simulink model "rede_PLL_Pcte_reativo"  (Simulink 7.8)
settings: Solver=ode3  StartTime=0.0  StopTime=3  FixedStep=1e-3  MaxStep=1e-3  RelTol=1e-3
libraries: powerlib_extras x5, simulink_need_slupdate x2, simulink x1, simulink_extras x1
settings Model: Creator=Batlab  LastModifiedBy=lgalotto
settings OptimizationCC: InitFltsAndDblsToZero=on
settings DebuggingCC: SaveWithParameterizedLinksMsg=none  FcnCallInpInsideContextMsg=Use local settings  StrictBusMsg=Warning
settings GRTTargetCC: TargetFcnLib=ansi_tfl_tmw.mat

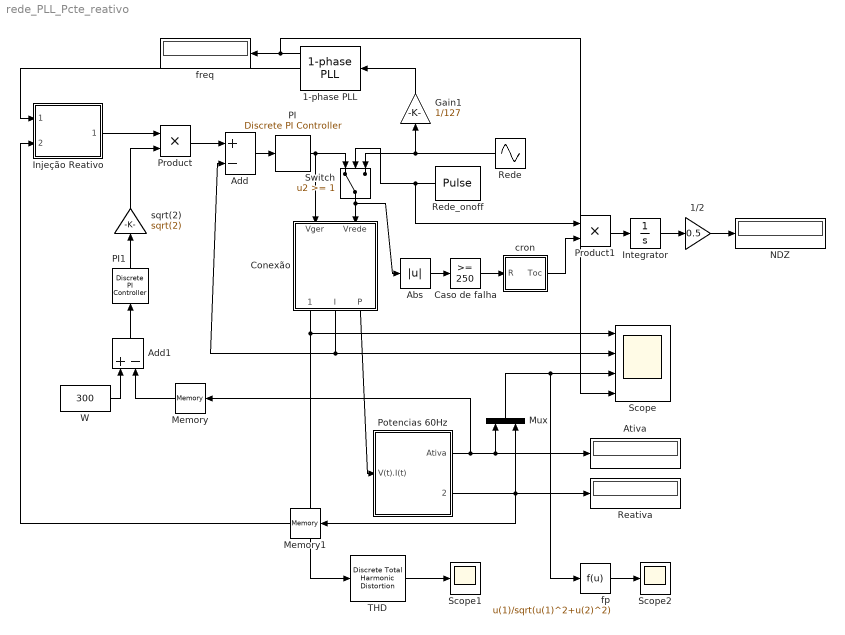
== system rede_PLL_Pcte_reativo ==
  1-phase PLL : powerlib_extras/Control  Blocks/1-phase PLL  Par_Init=[0 60]  ParK=[ 180 3200 1 ]  AGC=off
  1/2 : Gain  Gain=0.5
  Abs : Abs
  Add : Sum  Inputs=+-
  Add1 : Sum  Inputs=+-
  Ativa : Display
  Caso de falha : simulink/Logic and Bit Operations/Compare To Constant  relop=>=  const=250  OutDataTypeStr=uint8  ZeroCross=off
  Conexão : Subsystem
  Gain1 : Gain  Gain=1/127
  Injeção Reativo : Subsystem
  Integrator : Integrator
  Memory : Memory
  Memory1 : Memory
  Mux : Mux  Inputs=2
  NDZ : Display
  PI : powerlib_extras/Discrete  Control Blocks/Discrete PI Controller  Kp=10  Ki=20  Par_Limits=[1e3 -1e3]  Init=0  Ts=1e-3
  PI1 : powerlib_extras/Discrete  Control Blocks/Discrete PI Controller  Kp=0.02  Ki=0.08  Par_Limits=[40 0]  Init=10  Ts=1e-3
  Potencias 60Hz : Subsystem
  Product : Product  RndMeth=Zero
  Product1 : Product  RndMeth=Zero
  Reativa : Display
  Rede : Sin  Amplitude=127*sqrt(2)  Frequency=60*2*pi  SampleTime=0
  Rede_onoff : DiscretePulseGenerator  PulseType=Time based  Amplitude=2  PulseWidth=50  PhaseDelay=-1
  Scope : Scope  NumInputPorts=4
      settings: TimeRange=3  YMin=-200~-40~-2000~-5  YMax=200~20~4000~5  SaveName=dados
  Scope1 : Scope
      settings: TimeRange=3  YMin=-0.3919229176860233  YMax=0.6751100907072167
  Scope2 : Scope
      settings: TimeRange=3  YMin=0.8797282547329597  YMax=1
  Switch : Switch  Threshold=1
  THD : powerlib_extras/Discrete Measurements/Discrete Total Harmonic Distortion  Freq=60  Ts=1e-3
  W : Constant  Value=300
  cron : Subsystem
  fp : Fcn  Expr=u(1)/sqrt(u(1)^2+u(2)^2)
  freq : Display
  sqrt(2) : Gain  Gain=sqrt(2)
  wires:
  Conexão/1(Tensões) -> Scope/1, THD/1
  Conexão/3(P) -> Potencias 60Hz/1(V(t).I(t))
  Potencias 60Hz/2(Reativa) -> Reativa/1, Mux/2, Memory1/1
  Potencias 60Hz/1(Ativa) -> Ativa/1, Mux/1, Memory/1
  Conexão/2(I) -> Scope/2, Add/2
  Switch/1 -> Conexão/2(Vrede), Abs/1
  Rede/1 -> Gain1/1, Switch/3
  1-phase PLL/1 -> freq/1, Scope/4
  Gain1/1 -> 1-phase PLL/1
  Injeção Reativo/1(Ref. Corrente) -> Product/1
  Rede_onoff/1 -> Switch/2, Product1/1
  Product/1 -> Add/1
  Add/1 -> PI/1
  Mux/1 -> Scope/3, fp/1
  sqrt(2)/1 -> Product/2
  Add1/1 -> PI1/1
  PI1/1 -> sqrt(2)/1
  W/1 -> Add1/1
  Memory/1 -> Add1/2
  PI/1 -> Switch/1, Conexão/1(Vger)
  Memory1/1 -> Injeção Reativo/2(Reativo Medido)
  1-phase PLL/2 -> Injeção Reativo/1(wt_PLL)
  Abs/1 -> Caso de falha/1
  Caso de falha/1 -> cron/1(R)
  cron/1(Toc) -> Product1/2
  Integrator/1 -> 1/2/1
  1/2/1 -> NDZ/1
  Product1/1 -> Integrator/1
  THD/1 -> Scope1/1
  fp/1 -> Scope2/1

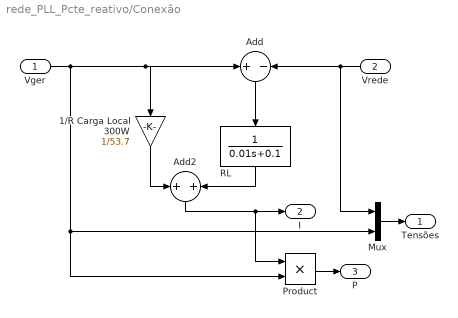
== system rede_PLL_Pcte_reativo/Conexão ==
  Vger : Inport
  Vrede : Inport  Port=2
  1/R Carga Local 300W : Gain  Gain=1/53.7
  Add : Sum  Inputs=+-
  Add2 : Sum  Inputs=2
  Mux : Mux  Inputs=2
  Product : Product  RndMeth=Zero
  RL : TransferFcn  Denominator=[0.01 0.1]
  Tensões : Outport
  I : Outport  Port=2
  P : Outport  Port=3
  wires:
  Vrede/1 -> Mux/1, Add/2
  Add/1 -> RL/1
  Vger/1 -> Product/2, Mux/2, Add/1, 1/R Carga Local 300W/1
  Mux/1 -> Tensões/1
  Product/1 -> P/1
  1/R Carga Local 300W/1 -> Add2/1
  Add2/1 -> I/1, Product/1
  RL/1 -> Add2/2

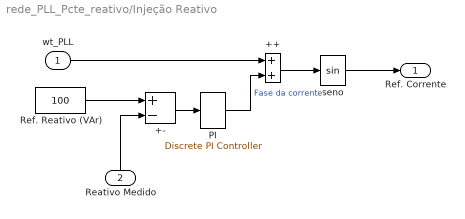
== system rede_PLL_Pcte_reativo/Injeção Reativo ==
  wt_PLL : Inport
  Reativo Medido : Inport  Port=2
  ++ : Sum  Inputs=2
  +- : Sum  Inputs=+-
  PI : powerlib_extras/Discrete  Control Blocks/Discrete PI Controller  Kp=0.001  Ki=0.02  Par_Limits=[1 -1]  Init=0  Ts=1e-3
  Ref. Reativo (VAr) : Constant  Value=100
  seno : Trigonometry
  Ref. Corrente : Outport
  wires:
  Ref. Reativo (VAr)/1 -> +-/1
  +-/1 -> PI/1
  ++/1 -> seno/1
  PI/1 -> ++/2  "Fase da corrente"
  wt_PLL/1 -> ++/1
  seno/1 -> Ref. Corrente/1
  Reativo Medido/1 -> +-/2

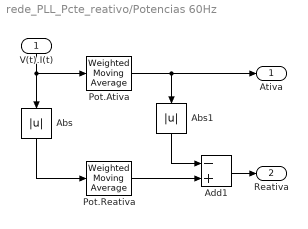
== system rede_PLL_Pcte_reativo/Potencias 60Hz ==
  V(t).I(t) : Inport
  Abs : Abs
  Abs1 : Abs
  Add1 : Sum  Inputs=-+
  Pot.Ativa : simulink_need_slupdate/Weighted Moving Average  mgainval=[ones(1,16)]./16  vinit=0.0  samptime=-1  OutDataType=sfix(16)  OutScaling=2^-10  DoSatur=off  GainDataType=sfix( 16 )  MatRadixGroup=Best Precision: Matrix-wise  GainScaling=2^-10
  Pot.Reativa : simulink_need_slupdate/Weighted Moving Average  mgainval=[ones(1,16)]./16  vinit=0.0  samptime=-1  OutDataType=sfix(16)  OutScaling=2^-10  DoSatur=off  GainDataType=sfix( 16 )  MatRadixGroup=Best Precision: Matrix-wise  GainScaling=2^-10
  Ativa : Outport
  Reativa : Outport  Port=2
  wires:
  Abs/1 -> Pot.Reativa/1
  Pot.Reativa/1 -> Add1/2
  Pot.Ativa/1 -> Abs1/1, Ativa/1
  Abs1/1 -> Add1/1
  V(t).I(t)/1 -> Abs/1, Pot.Ativa/1
  Add1/1 -> Reativa/1

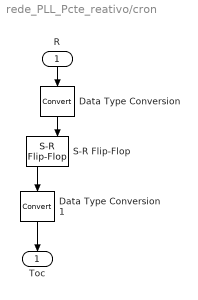
== system rede_PLL_Pcte_reativo/cron ==
  R : Inport
  Data Type Conversion : DataTypeConversion
  Data Type Conversion1 : DataTypeConversion
  S-R Flip-Flop : simulink_extras/Flip Flops/S-R Flip-Flop  initial_condition=1
  Toc : Outport
  wires:
  R/1 -> Data Type Conversion/1
  S-R Flip-Flop/1 -> Data Type Conversion1/1
  Data Type Conversion/1 -> S-R Flip-Flop/2
  Data Type Conversion1/1 -> Toc/1
